simulink model "sim_3"  (R2021b)
settings: Solver=FixedStepAuto  StartTime=0.0  StopTime=100  FixedStep=0.01  RelTol=1e-3
values from neighbouring files (symbols this model uses):
  lambda0 = tc.lambda0_tc    [gnrt_tc.m]
  r0 = tc.r0_tc    [gnrt_tc.m]
  v_lam0 = tc.v_lam0_tc    [gnrt_tc.m]
  v_r0 = tc.v_r0_tc    [gnrt_tc.m]
  zeta = tc.zeta_tc    [gnrt_tc.m]
libraries: simulink x1
settings Model: Creator=kusha  LastModifiedBy=kusha

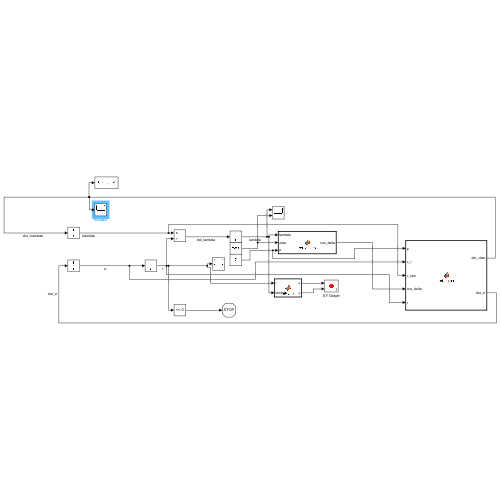
[thumbnail: Simulink's stored preview of the top-level diagram]
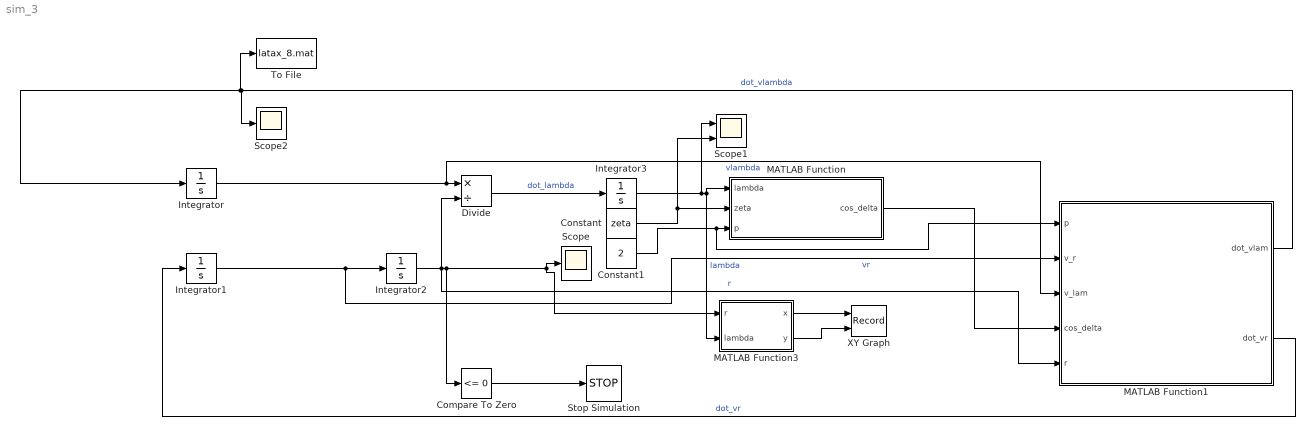
== system sim_3 ==
  Compare To Zero : simulink/Logic and Bit Operations/Compare To Zero  relop=<=  OutDataTypeStr=boolean
  Constant : Constant  Value=zeta
  Constant1 : Constant  Value=2
  Divide : Product  Inputs=*/
  Integrator : Integrator  InitialCondition=v_lam0
  Integrator1 : Integrator  InitialCondition=v_r0
  Integrator2 : Integrator  InitialCondition=r0
  Integrator3 : Integrator  InitialCondition=lambda0
  MATLAB Function : MATLAB Function  TreatAsAtomicUnit=on
  MATLAB Function1 : MATLAB Function  TreatAsAtomicUnit=on
  MATLAB Function3 : MATLAB Function  TreatAsAtomicUnit=on
  Scope : Scope
  Scope1 : Scope  NumInputPorts=2
  Scope2 : Scope
  Stop Simulation : Stop
  To File : ToFile  Filename=latax_8.mat  SaveFormat=Timeseries
  XY Graph : Record  FileSettingsInternal="{\"entries\":[{\"content\":{\"excelSettings\":{\"content\":{},\"type\":\"Streamout.ExcelSettings\"}},\"type\":\"Streamout.FileSettingStorage\",\"uuid\":\"7a2c49ac-6534-4055-b3dc-b3cdbea7ba03\"}],\"packageUris\":[\"http://schema.mathworks.com/mf0/streamout_blocks/R2020a\"],\"version\":\"1.0\"}"  Layout=[1 1]  SignalsInternal="{\"entries\":[{\"content\":{\"signals\":[{\"content\":{\"blockPath\":[\"sim_3/XY Graph\"],\"channel\":[],\"dimensions\":[1],\"domain\":\"sim_3/XY Graph\",\"lineColor\":\"#a2142f\",\"plots\":[1],\"port\":1,\"sid\":[\"\"],\"signalID\":417,\"signalName\":\"MATLAB Function3:1\"},\"type\":\"RecordBlkView.Signal\",\"uuid\":\"e8995922-1af0-4153-bbdd-969861f5b825\"},{\"content\":{\"blockPath\":[\"sim_3/XY Graph\"],\"channel\":[],\"dimensions\":[1],\"domain\":\"sim_3/XY Graph\",\"lineColor\":\"#139fff\",\"plots\":[1],\"port\":2,\"sid\":[\"\"],\"signalID\":421,\"signalName\":\"MATLAB Function3:2\"},\"type\":\"RecordBlkView.Signal\",\"uuid\":\"d4577de4-4bfc-480d-b094-fd1fee2f6386\"}]},\"type\":\"RecordBlkView.InputSignals\",\"uuid\":\"e729227f-bef8-4fcc-8143-819f1af59332\"}],\"packageUris\":[\"http://schema.mathworks.com/mf0/streamout_blocks/R2020a\"],\"version\":\"1.0\"}"  VisualizationBindings="{\"xyplotplugin\":{\"info\":[{\"series\":[{\"bindingParametersList\":[{\"parameter\":\"X-Axis\",\"signalID\":417,\"signalName\":\"MATLAB Function3:1\"},{\"parameter\":\"Y-Axis\",\"signalID\":421,\"signalName\":\"MATLAB Function3:2\"}],\"seriesID\":43248}],\"subplotID\":1}]}}"  CompatibilityTag=XY
  wires:
  Compare To Zero/1 -> Stop Simulation/1
  Integrator2/1 -> Divide/2, Compare To Zero/1, MATLAB Function3/1(r), Scope/1, MATLAB Function1/5(r)  "r"
  MATLAB Function3/1(x) -> XY Graph/1
  MATLAB Function3/2(y) -> XY Graph/2
  MATLAB Function1/1(dot_vlam) -> Scope2/1, To File/1, Integrator/1  "dot_vlambda"
  Constant/1 -> MATLAB Function/2(zeta), Scope1/2
  MATLAB Function/1(cos_delta) -> MATLAB Function1/4(cos_delta)
  MATLAB Function1/2(dot_vr) -> Integrator1/1  "dot_vr"
  Integrator/1 -> MATLAB Function1/3(v_lam), Divide/1  "vlambda"
  Integrator1/1 -> MATLAB Function1/2(v_r), Integrator2/1  "vr"
  Divide/1 -> Integrator3/1  "dot_lambda"
  Integrator3/1 -> Scope1/1, MATLAB Function3/2(lambda), MATLAB Function/1(lambda)  "lambda"
  Constant1/1 -> MATLAB Function1/1(p), MATLAB Function/3(p)

== matlab function sim_3/MATLAB Function1 ==
  data: p input; v_r input; dot_vlam output; v_lam input; cos_delta input; r input; dot_vr output
function [dot_vlam, dot_vr] = ret_rates(p, v_r, v_lam, cos_delta, r)
dot_vlam = 1/p*v_r*v_lam*(cos_delta^2)/r;
dot_vr = -1/p*(v_lam^2)*(cos_delta^2)/r;

== matlab function sim_3/MATLAB Function ==
  data: lambda input; cos_delta output; zeta input; p input
function cos_delta = ret_deltap(lambda, zeta, p)

delta = atan(1/p*(lambda - zeta));
cos_delta = cos(delta);

== matlab function sim_3/MATLAB Function3 ==
  data: x output; r input; y output; lambda input
function [x, y] = ret_x_y(r, lambda)

x = r*cos(lambda);
y = r*sin(lambda);
